simulink library "sm_rollerV_lib_terrain_contact_r9"  (R2026a)
settings: Solver=VariableStepAuto
undefined symbols (not defined in the file): B1, B2, B3, B4, B5, B6, B7, B8, P1, P2, P3, P4, P5, P6, P7, P8, P9, Road, Scene, X, Y, Z
libraries: $bdroot x19, sm_trackV_lib_terrain_contact_elem x18, sm_excv_scene_lib x4, sm_lib x4
Description:
  | Copyright 2024-2026 The MathWorks, Inc.
settings Model: Creator=smiller  LastModifiedBy=smiller

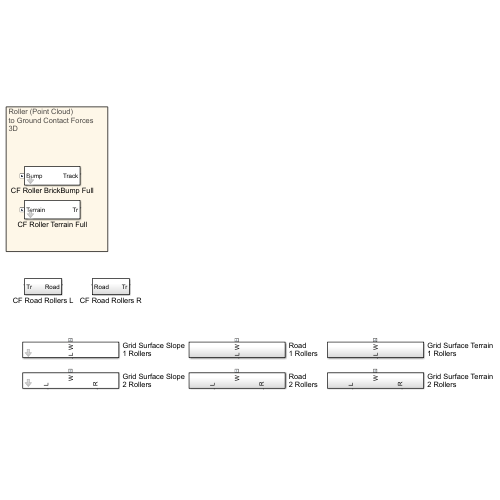
[thumbnail: Simulink's stored preview of the top-level diagram]
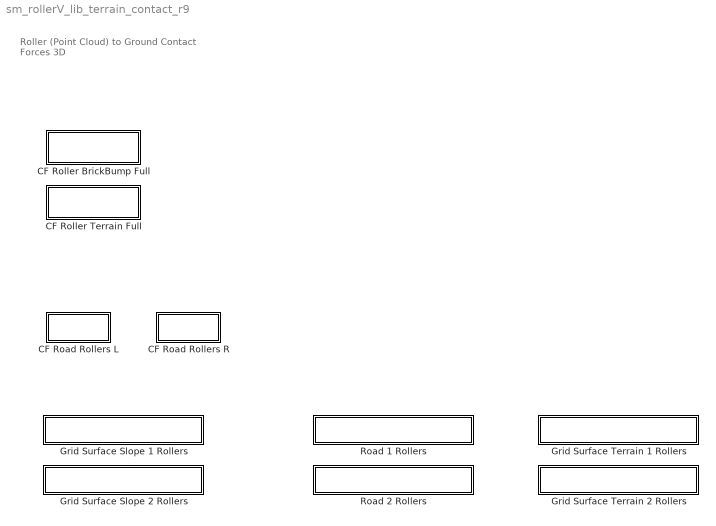
== system sm_rollerV_lib_terrain_contact_r9 ==
  note: Roller (Point Cloud)
      | to Ground Contact Forces
      | 3D
  CF Road Rollers L : Subsystem
  CF Road Rollers R : Subsystem
  CF Roller BrickBump Full : Subsystem  mask(Contact Forces, Rollers to Bump){K_BrickBump=Scene.Contact.BrickBump.K, B_BrickBump=Scene.Contact.BrickBump.B, TW_BrickBump=Scene.Contact.BrickBump.TW}
      mask prompts: K_BrickBump "Normal Stiffness (N/m)"; B_BrickBump "Normal Damping (N/(m/s))"; TW_BrickBump "Normal Transition Width (m)"
      mask help: Models contact force between rolling elements and bump.
  CF Roller Terrain Full : Subsystem  mask(Contact Forces, Rollers to Terrain){K_Road=Scene.Contact.Terrain.K, B_Road=Scene.Contact.Terrain.B, TW_Road=Scene.Contact.Terrain.TW, F_dyn_Road=Scene.Contact.Terrain.mud, F_stat_Road=Scene.Contact.Terrain.mus, CV_Road=Scene.Contact.Terrain.CV}
      mask prompts: K_Road "Normal Stiffness (N/m)"; B_Road "Normal Damping (N/(m/s))"; TW_Road "Normal Transition Width (m)"; F_dyn_Road "Coefficient of Dynamic Friction"; F_stat_Road "Coefficient of Static Friction"; CV_Road "Critical Velocity (m/s)"
      mask help: Models contact force between rolling elements and terrain.
  Grid Surface Slope 1 Rollers : Subsystem  mask{road_len=Scene.Slope.road_len, road_wid=Scene.Slope.road_wid, slope_rise=Scene.Slope.slope_rise, slope_run=Scene.Slope.slope_run, slope_x0=Scene.Slope.slope_start, slope_xres=Scene.Slope.slope_xres, surface_clr=Scene.Slope.clr, surface_opc=Scene.Slope.opc, K_Road=Scene.Contact.Terrain.K, B_Road=Scene.Contact.Terrain.B, TW_Road=Scene.Contact.Terrain.TW, F_dyn_Road=Scene.Contact.Terrain.mud, F_stat_Road=Scene.Contact.Terrain.mus, CV_Road=Scene.Contact.Terrain.CV}
      mask prompts: road_len "Road Length (m)"; road_wid "Road Width (m)"; slope_rise "Slope Rise (m)"; slope_run "Slope Run(m)"; slope_x0 "Slope Start (m)"; slope_xres "Slope Resolution (m)"; surface_clr "Color [R G B] (0-1)"; surface_opc "Opacity (0-1)"; K_Road "Normal Stiffness (N/m)"; B_Road "Normal Damping (N/(m/s))"; TW_Road "Normal Transition Width (m)"; F_dyn_Road "Coefficient of Dynamic Friction"; F_stat_Road "Coefficient of Static Friction"; CV_Road "Critical Velocity (m/s)"
      mask TypeOptions road_len:
      | Grid Surface
      | Slope/road_len
      mask TypeOptions road_wid:
      | Grid Surface
      | Slope/road_wid
      mask TypeOptions slope_rise:
      | Grid Surface
      | Slope/slope_rise
      mask TypeOptions slope_run:
      | Grid Surface
      | Slope/slope_run
      mask TypeOptions slope_x0:
      | Grid Surface
      | Slope/slope_x0
      mask TypeOptions slope_xres:
      | Grid Surface
      | Slope/slope_xres
      mask TypeOptions surface_clr:
      | Grid Surface
      | Slope/surface_clr
      mask TypeOptions surface_opc:
      | Grid Surface
      | Slope/surface_opc
      mask TypeOptions K_Road: CF Track Terrain L/K_Road
      mask TypeOptions B_Road: CF Track Terrain L/B_Road
      mask TypeOptions TW_Road: CF Track Terrain L/TW_Road
      mask TypeOptions F_dyn_Road: CF Track Terrain L/F_dyn_Road
      mask TypeOptions F_stat_Road: CF Track Terrain L/F_stat_Road
      mask TypeOptions CV_Road: CF Track Terrain L/CV_Road
      mask DialogControl cont_slope Prompt: Slope
      mask DialogControl cont_contact Prompt: Contact
  Grid Surface Slope 2 Rollers : Subsystem  mask{road_len=Scene.Slope.road_len, road_wid=Scene.Slope.road_wid, slope_rise=Scene.Slope.slope_rise, slope_run=Scene.Slope.slope_run, slope_x0=Scene.Slope.slope_start, slope_xres=Scene.Slope.slope_xres, surface_clr=Scene.Slope.clr, surface_opc=Scene.Slope.opc, K_Road=Scene.Contact.Terrain.K, B_Road=Scene.Contact.Terrain.B, TW_Road=Scene.Contact.Terrain.TW, F_dyn_Road=Scene.Contact.Terrain.mud, F_stat_Road=Scene.Contact.Terrain.mus, CV_Road=Scene.Contact.Terrain.CV}
      mask prompts: road_len "Road Length (m)"; road_wid "Road Width (m)"; slope_rise "Slope Rise (m)"; slope_run "Slope Run(m)"; slope_x0 "Slope Start (m)"; slope_xres "Slope Resolution (m)"; surface_clr "Color [R G B] (0-1)"; surface_opc "Opacity (0-1)"; K_Road "Normal Stiffness (N/m)"; B_Road "Normal Damping (N/(m/s))"; TW_Road "Normal Transition Width (m)"; F_dyn_Road "Coefficient of Dynamic Friction"; F_stat_Road "Coefficient of Static Friction"; CV_Road "Critical Velocity (m/s)"
      mask TypeOptions road_len:
      | Grid Surface
      | Slope/road_len
      mask TypeOptions road_wid:
      | Grid Surface
      | Slope/road_wid
      mask TypeOptions slope_rise:
      | Grid Surface
      | Slope/slope_rise
      mask TypeOptions slope_run:
      | Grid Surface
      | Slope/slope_run
      mask TypeOptions slope_x0:
      | Grid Surface
      | Slope/slope_x0
      mask TypeOptions slope_xres:
      | Grid Surface
      | Slope/slope_xres
      mask TypeOptions surface_clr:
      | Grid Surface
      | Slope/surface_clr
      mask TypeOptions surface_opc:
      | Grid Surface
      | Slope/surface_opc
      mask TypeOptions K_Road: CF Track Terrain L/K_Road
      mask TypeOptions B_Road: CF Track Terrain L/B_Road
      mask TypeOptions TW_Road: CF Track Terrain L/TW_Road
      mask TypeOptions F_dyn_Road: CF Track Terrain L/F_dyn_Road
      mask TypeOptions F_stat_Road: CF Track Terrain L/F_stat_Road
      mask TypeOptions CV_Road: CF Track Terrain L/CV_Road
      mask DialogControl cont_slope Prompt: Slope
      mask DialogControl cont_contact Prompt: Contact
  Grid Surface Terrain 1 Rollers : Subsystem
  Grid Surface Terrain 2 Rollers : Subsystem
  Road 1 Rollers : Subsystem
  Road 2 Rollers : Subsystem

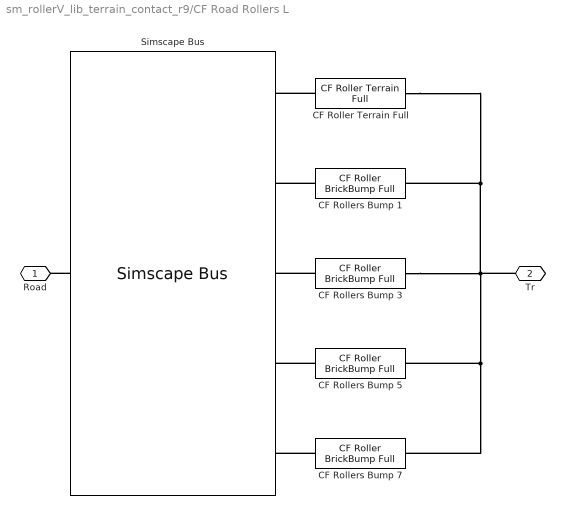
== system sm_rollerV_lib_terrain_contact_r9/CF Road Rollers L ==
  CF Roller Terrain Full : $bdroot/CF Roller Terrain Full  K_Road=Scene.Contact.Terrain.K  B_Road=Scene.Contact.Terrain.B  TW_Road=Scene.Contact.Terrain.TW  F_dyn_Road=Scene.Contact.Terrain.mud  F_stat_Road=Scene.Contact.Terrain.mus  CV_Road=Scene.Contact.Terrain.CV
  "CF Rollers Bump 1 " : $bdroot/CF Roller BrickBump Full  K_BrickBump=Scene.Contact.BrickBump.K  B_BrickBump=Scene.Contact.BrickBump.B  TW_BrickBump=Scene.Contact.BrickBump.TW
  CF Rollers Bump 3 : $bdroot/CF Roller BrickBump Full  K_BrickBump=Scene.Contact.BrickBump.K  B_BrickBump=Scene.Contact.BrickBump.B  TW_BrickBump=Scene.Contact.BrickBump.TW
  CF Rollers Bump 5 : $bdroot/CF Roller BrickBump Full  K_BrickBump=Scene.Contact.BrickBump.K  B_BrickBump=Scene.Contact.BrickBump.B  TW_BrickBump=Scene.Contact.BrickBump.TW
  CF Rollers Bump 7 : $bdroot/CF Roller BrickBump Full  K_BrickBump=Scene.Contact.BrickBump.K  B_BrickBump=Scene.Contact.BrickBump.B  TW_BrickBump=Scene.Contact.BrickBump.TW
  Simscape Bus : SimscapeBus  HierarchyStrings=Road;B1;B3;B5;B7  ConnectionType=Bus: CBO_Road8
  Road : PMIOPort  Side=Left
  Tr : PMIOPort  Port=2  Side=Right
  connections:
  CF Rollers Bump 7/RConn1 -- CF Rollers Bump 5/RConn1 -- "CF Rollers Bump 1 "/RConn1 -- CF Roller Terrain Full/RConn1 -- CF Rollers Bump 3/RConn1 -- Tr/RConn1
  CF Rollers Bump 7/LConn1 -- Simscape Bus/LConn5
  CF Rollers Bump 5/LConn1 -- Simscape Bus/LConn4
  Simscape Bus/RConn1 -- Road/RConn1
  CF Roller Terrain Full/LConn1 -- Simscape Bus/LConn1
  "CF Rollers Bump 1 "/LConn1 -- Simscape Bus/LConn2
  CF Rollers Bump 3/LConn1 -- Simscape Bus/LConn3

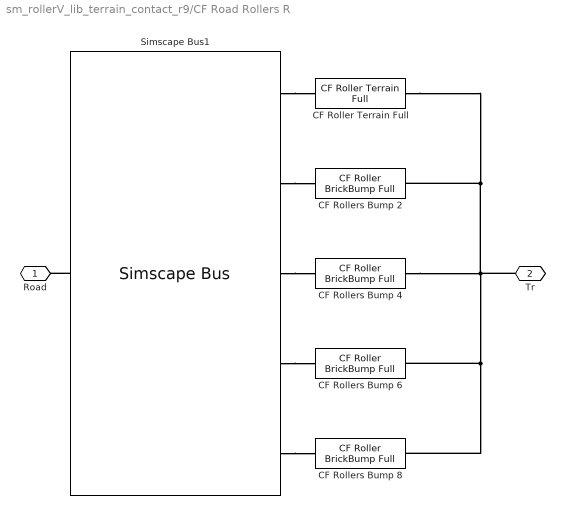
== system sm_rollerV_lib_terrain_contact_r9/CF Road Rollers R ==
  CF Roller Terrain Full : $bdroot/CF Roller Terrain Full  K_Road=Scene.Contact.Terrain.K  B_Road=Scene.Contact.Terrain.B  TW_Road=Scene.Contact.Terrain.TW  F_dyn_Road=Scene.Contact.Terrain.mud  F_stat_Road=Scene.Contact.Terrain.mus  CV_Road=Scene.Contact.Terrain.CV
  "CF Rollers Bump 2 " : $bdroot/CF Roller BrickBump Full  K_BrickBump=Scene.Contact.BrickBump.K  B_BrickBump=Scene.Contact.BrickBump.B  TW_BrickBump=Scene.Contact.BrickBump.TW
  CF Rollers Bump 4 : $bdroot/CF Roller BrickBump Full  K_BrickBump=Scene.Contact.BrickBump.K  B_BrickBump=Scene.Contact.BrickBump.B  TW_BrickBump=Scene.Contact.BrickBump.TW
  CF Rollers Bump 6 : $bdroot/CF Roller BrickBump Full  K_BrickBump=Scene.Contact.BrickBump.K  B_BrickBump=Scene.Contact.BrickBump.B  TW_BrickBump=Scene.Contact.BrickBump.TW
  CF Rollers Bump 8 : $bdroot/CF Roller BrickBump Full  K_BrickBump=Scene.Contact.BrickBump.K  B_BrickBump=Scene.Contact.BrickBump.B  TW_BrickBump=Scene.Contact.BrickBump.TW
  Simscape Bus1 : SimscapeBus  HierarchyStrings=Road;B2;B4;B6;B8  ConnectionType=Bus: CBO_Road8
  Road : PMIOPort  Side=Left
  Tr : PMIOPort  Port=2  Side=Right
  connections:
  Simscape Bus1/LConn3 -- CF Rollers Bump 4/LConn1
  Simscape Bus1/LConn2 -- "CF Rollers Bump 2 "/LConn1
  Simscape Bus1/LConn1 -- CF Roller Terrain Full/LConn1
  Simscape Bus1/RConn1 -- Road/RConn1
  Simscape Bus1/LConn4 -- CF Rollers Bump 6/LConn1
  Simscape Bus1/LConn5 -- CF Rollers Bump 8/LConn1
  CF Rollers Bump 4/RConn1 -- Tr/RConn1 -- CF Rollers Bump 6/RConn1 -- CF Rollers Bump 8/RConn1 -- "CF Rollers Bump 2 "/RConn1 -- CF Roller Terrain Full/RConn1

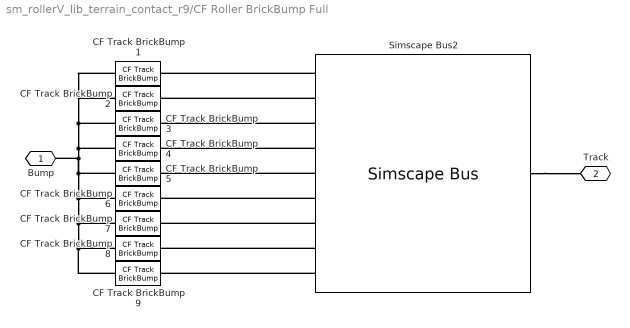
== system sm_rollerV_lib_terrain_contact_r9/CF Roller BrickBump Full ==
  CF Track BrickBump {1..9} (9 alike) : sm_trackV_lib_terrain_contact_elem/CF Track BrickBump  NormalStiffness=K_BrickBump  NormalDamping=B_BrickBump  NormalTransitionRegionWidth=TW_BrickBump
      settings: LibrarySourceBlock=sm_chain_drive_lib/CF_BrickBump
  Simscape Bus2 : SimscapeBus  HierarchyStrings=P1;P2;P3;P4;P5;P6;P7;P8;P9  ConnectionType=Bus: CBO_Roller9
  Bump : PMIOPort  Side=Left
  Track : PMIOPort  Port=2  Side=Right
  connections:
  CF Track BrickBump 6/LConn1 -- CF Track BrickBump 7/LConn1 -- CF Track BrickBump 8/LConn1 -- CF Track BrickBump 9/LConn1 -- Bump/RConn1 -- CF Track BrickBump 1/LConn1 -- CF Track BrickBump 2/LConn1 -- CF Track BrickBump 3/LConn1 -- CF Track BrickBump 4/LConn1 -- CF Track BrickBump 5/LConn1
  Simscape Bus2/RConn1 -- Track/RConn1
  Simscape Bus2/LConn1 -- CF Track BrickBump 1/RConn1
  Simscape Bus2/LConn2 -- CF Track BrickBump 2/RConn1
  Simscape Bus2/LConn4 -- CF Track BrickBump 4/RConn1
  Simscape Bus2/LConn3 -- CF Track BrickBump 3/RConn1
  Simscape Bus2/LConn5 -- CF Track BrickBump 5/RConn1
  Simscape Bus2/LConn6 -- CF Track BrickBump 6/RConn1
  Simscape Bus2/LConn7 -- CF Track BrickBump 7/RConn1
  Simscape Bus2/LConn8 -- CF Track BrickBump 8/RConn1
  Simscape Bus2/LConn9 -- CF Track BrickBump 9/RConn1

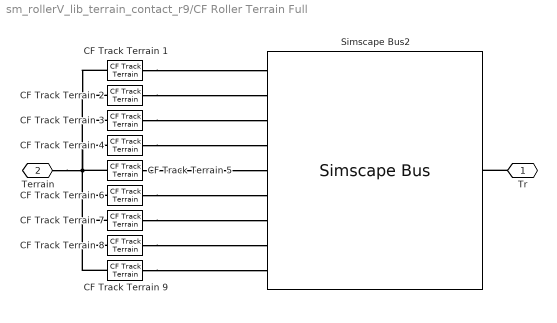
== system sm_rollerV_lib_terrain_contact_r9/CF Roller Terrain Full ==
  CF Track Terrain {1..9} (9 alike) : sm_trackV_lib_terrain_contact_elem/CF Track Terrain  NormalStiffness=K_Road  NormalDamping=B_Road  NormalTransitionRegionWidth=TW_Road  CoefficientOfDynamicFriction=F_dyn_Road  CoefficientOfStaticFriction=F_stat_Road  FrictionalCriticalVelocity=CV_Road
      settings: LibrarySourceBlock=sm_chain_drive_lib/CF_Road
  Simscape Bus2 : SimscapeBus  HierarchyStrings=P1;P2;P3;P4;P5;P6;P7;P8;P9  ConnectionType=Bus: CBO_Roller9
  Tr : PMIOPort  Side=Right
  Terrain : PMIOPort  Port=2  Side=Left
  connections:
  CF Track Terrain 9/RConn1 -- Simscape Bus2/LConn9
  CF Track Terrain 1/LConn1 -- CF Track Terrain 2/LConn1 -- CF Track Terrain 3/LConn1 -- CF Track Terrain 4/LConn1 -- CF Track Terrain 5/LConn1 -- CF Track Terrain 6/LConn1 -- CF Track Terrain 7/LConn1 -- CF Track Terrain 9/LConn1 -- CF Track Terrain 8/LConn1 -- Terrain/RConn1
  CF Track Terrain 8/RConn1 -- Simscape Bus2/LConn8
  CF Track Terrain 3/RConn1 -- Simscape Bus2/LConn3
  CF Track Terrain 2/RConn1 -- Simscape Bus2/LConn2
  CF Track Terrain 1/RConn1 -- Simscape Bus2/LConn1
  CF Track Terrain 7/RConn1 -- Simscape Bus2/LConn7
  CF Track Terrain 5/RConn1 -- Simscape Bus2/LConn5
  CF Track Terrain 4/RConn1 -- Simscape Bus2/LConn4
  CF Track Terrain 6/RConn1 -- Simscape Bus2/LConn6
  Tr/RConn1 -- Simscape Bus2/RConn1

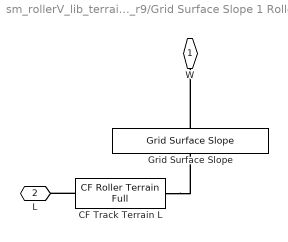
== system sm_rollerV_lib_terrain_contact_r9/Grid Surface Slope 1 Rollers ==
  CF Track Terrain L : $bdroot/CF Roller Terrain Full  K_Road=K_Road  B_Road=B_Road  TW_Road=TW_Road  F_dyn_Road=F_dyn_Road  F_stat_Road=F_stat_Road  CV_Road=CV_Road
  Grid Surface Slope : sm_excv_scene_lib/Grid Surface Slope  road_len=road_len  road_wid=road_wid  slope_run=slope_run  slope_rise=slope_rise  slope_x0=slope_x0  slope_xres=slope_xres  surface_clr=surface_clr  surface_opc=surface_opc
  W : PMIOPort  Side=Right
  L : PMIOPort  Port=2  Side=Left
  connections:
  CF Track Terrain L/RConn1 -- L/RConn1
  Grid Surface Slope/RConn1 -- W/RConn1
  CF Track Terrain L/LConn1 -- Grid Surface Slope/LConn1

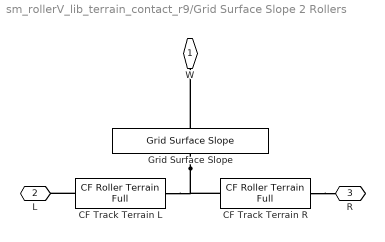
== system sm_rollerV_lib_terrain_contact_r9/Grid Surface Slope 2 Rollers ==
  CF Track Terrain L : $bdroot/CF Roller Terrain Full  K_Road=K_Road  B_Road=B_Road  TW_Road=TW_Road  F_dyn_Road=F_dyn_Road  F_stat_Road=F_stat_Road  CV_Road=CV_Road
  CF Track Terrain R : $bdroot/CF Roller Terrain Full  K_Road=K_Road  B_Road=B_Road  TW_Road=TW_Road  F_dyn_Road=F_dyn_Road  F_stat_Road=F_stat_Road  CV_Road=CV_Road
  Grid Surface Slope : sm_excv_scene_lib/Grid Surface Slope  road_len=road_len  road_wid=road_wid  slope_run=slope_run  slope_rise=slope_rise  slope_x0=slope_x0  slope_xres=slope_xres  surface_clr=surface_clr  surface_opc=surface_opc
  W : PMIOPort  Side=Right
  L : PMIOPort  Port=2  Side=Left
  R : PMIOPort  Port=3  Side=Left
  connections:
  CF Track Terrain R/RConn1 -- R/RConn1
  Grid Surface Slope/LConn1 -- CF Track Terrain R/LConn1 -- CF Track Terrain L/LConn1
  Grid Surface Slope/RConn1 -- W/RConn1
  CF Track Terrain L/RConn1 -- L/RConn1

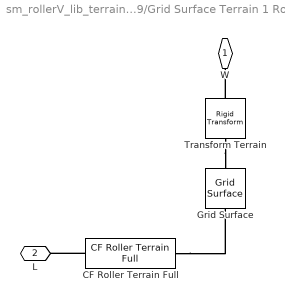
== system sm_rollerV_lib_terrain_contact_r9/Grid Surface Terrain 1 Rollers ==
  CF Roller Terrain Full : $bdroot/CF Roller Terrain Full  K_Road=Scene.Contact.Terrain.K  B_Road=Scene.Contact.Terrain.B  TW_Road=Scene.Contact.Terrain.TW  F_dyn_Road=Scene.Contact.Terrain.mud  F_stat_Road=Scene.Contact.Terrain.mus  CV_Road=Scene.Contact.Terrain.CV
  Grid Surface : sm_lib/Curves and Surfaces/Grid Surface  XGridVector=Scene.Terrain.xg  XGridVectorUnits=m  YGridVector=Scene.Terrain.yg  YGridVectorUnits=m  ZHeights=Scene.Terrain.z_heights_data  ZHeightsUnits=m  GraphicType=FromGeometry  GraphicVisPropType=SimpleVisualProperties  GraphicDiffuseColor=[0.8196 0.7255 0.5098]  GraphicOpacity=1.0  GraphicSpecularColor=[0.5 0.5 0.5 1.0]  GraphicAmbientColor=[0.15 0.15 0.15 1.0]  GraphicEmissiveColor=[0.0 0.0 0.0 1.0]  GraphicShininess=75
  Transform Terrain : sm_lib/Frames and Transforms/Rigid Transform  RotationMethod=None  FollAlignAxisA=+X  BaseAlignAxisA=+Y  FollAlignAxisB=+Y  BaseAlignAxisB=+Z  RotationStandardAxis=+Z  RotationAngle=0.0  RotationAngleUnits=deg  RotationArbitraryAxis=[0 0 1]  RotationSequenceAxes=FollowerAxes  RotationSequence=XYX  RotationSequenceAngles=[0 0 0]  RotationSequenceAnglesUnits=deg  RotationMatrix=[1 0 0; 0 1 0; 0 0 1]  Quaternion=[1 0 0 0]  TranslationMethod=Cartesian  TranslationCartesianOffset="[-45 -45+2.5  -2.75+0.2]"  TranslationCartesianOffsetUnits=m  TranslationStandardAxis=+Z  TranslationStandardOffset=0  TranslationStandardOffsetUnits=m  TranslationROffset=0  TranslationROffsetUnits=m  TranslationThetaOffset=0  TranslationThetaOffsetUnits=deg  TranslationZOffset=0  TranslationZOffsetUnits=m
  W : PMIOPort  Side=Right
  L : PMIOPort  Port=2  Side=Left
  connections:
  CF Roller Terrain Full/RConn1 -- L/RConn1
  Transform Terrain/LConn1 -- W/RConn1
  CF Roller Terrain Full/LConn1 -- Grid Surface/RConn1
  Transform Terrain/RConn1 -- Grid Surface/LConn1

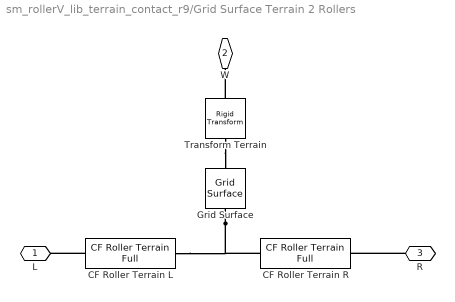
== system sm_rollerV_lib_terrain_contact_r9/Grid Surface Terrain 2 Rollers ==
  CF Roller Terrain L : $bdroot/CF Roller Terrain Full  K_Road=Scene.Contact.Terrain.K  B_Road=Scene.Contact.Terrain.B  TW_Road=Scene.Contact.Terrain.TW  F_dyn_Road=Scene.Contact.Terrain.mud  F_stat_Road=Scene.Contact.Terrain.mus  CV_Road=Scene.Contact.Terrain.CV
  CF Roller Terrain R : $bdroot/CF Roller Terrain Full  K_Road=Scene.Contact.Terrain.K  B_Road=Scene.Contact.Terrain.B  TW_Road=Scene.Contact.Terrain.TW  F_dyn_Road=Scene.Contact.Terrain.mud  F_stat_Road=Scene.Contact.Terrain.mus  CV_Road=Scene.Contact.Terrain.CV
  Grid Surface : sm_lib/Curves and Surfaces/Grid Surface  XGridVector=Scene.Terrain.xg  XGridVectorUnits=m  YGridVector=Scene.Terrain.yg  YGridVectorUnits=m  ZHeights=Scene.Terrain.z_heights_data  ZHeightsUnits=m  GraphicType=FromGeometry  GraphicVisPropType=SimpleVisualProperties  GraphicDiffuseColor=[0.8196 0.7255 0.5098]  GraphicOpacity=1.0  GraphicSpecularColor=[0.5 0.5 0.5 1.0]  GraphicAmbientColor=[0.15 0.15 0.15 1.0]  GraphicEmissiveColor=[0.0 0.0 0.0 1.0]  GraphicShininess=75
  Transform Terrain : sm_lib/Frames and Transforms/Rigid Transform  RotationMethod=None  FollAlignAxisA=+X  BaseAlignAxisA=+Y  FollAlignAxisB=+Y  BaseAlignAxisB=+Z  RotationStandardAxis=+Z  RotationAngle=0.0  RotationAngleUnits=deg  RotationArbitraryAxis=[0 0 1]  RotationSequenceAxes=FollowerAxes  RotationSequence=XYX  RotationSequenceAngles=[0 0 0]  RotationSequenceAnglesUnits=deg  RotationMatrix=[1 0 0; 0 1 0; 0 0 1]  Quaternion=[1 0 0 0]  TranslationMethod=Cartesian  TranslationCartesianOffset="[-45 -45+2.5  -2.75+0.2]"  TranslationCartesianOffsetUnits=m  TranslationStandardAxis=+Z  TranslationStandardOffset=0  TranslationStandardOffsetUnits=m  TranslationROffset=0  TranslationROffsetUnits=m  TranslationThetaOffset=0  TranslationThetaOffsetUnits=deg  TranslationZOffset=0  TranslationZOffsetUnits=m
  L : PMIOPort  Side=Left
  W : PMIOPort  Port=2  Side=Right
  R : PMIOPort  Port=3  Side=Left
  connections:
  R/RConn1 -- CF Roller Terrain R/RConn1
  Transform Terrain/RConn1 -- Grid Surface/LConn1
  Grid Surface/RConn1 -- CF Roller Terrain R/LConn1 -- CF Roller Terrain L/LConn1
  Transform Terrain/LConn1 -- W/RConn1
  CF Roller Terrain L/RConn1 -- L/RConn1

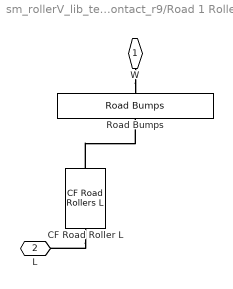
== system sm_rollerV_lib_terrain_contact_r9/Road 1 Rollers ==
  CF Road Roller L : $bdroot/CF Road Rollers L  SystemSampleTime=-1  VariantActivationTime=update diagram  EmptyChoice=off  PassThrough=off  PassThroughVariantControl=(default)  EmptyChoiceVariantControl=(default)  AllowFlexibleInterface=on  Latency=0  AutoFrameSizeCalculation=off
      settings: LibrarySourceBlock=|
      | sm_excv_scene_lib/CF
      | Road
      | Roller L
  Road Bumps : sm_excv_scene_lib/Road Bumps  road_x=Scene.Road.len  road_y=Scene.Road.wid  road_z=Scene.Road.hgt  bump_x=Scene.Road.Bump.len  bump_y=Scene.Road.Bump.wid  bump_z=Scene.Road.Bump.hgt  bloc_y=Scene.Road.Bump.offsety  bloc_z=Scene.Road.Bump.offsetz  bump_x0=Scene.Road.Bump.startx  bloc_dx=Scene.Road.Bump.deltax
  W : PMIOPort  Side=Right
  L : PMIOPort  Port=2  Side=Left
  connections:
  CF Road Roller L/RConn1 -- L/RConn1
  CF Road Roller L/LConn1 -- Road Bumps/LConn1
  W/RConn1 -- Road Bumps/RConn1

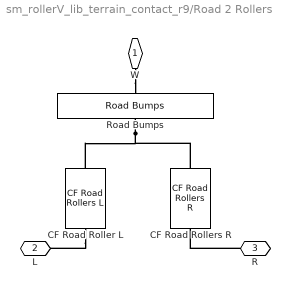
== system sm_rollerV_lib_terrain_contact_r9/Road 2 Rollers ==
  CF Road Roller L : $bdroot/CF Road Rollers L  SystemSampleTime=-1  VariantActivationTime=update diagram  EmptyChoice=off  PassThrough=off  PassThroughVariantControl=(default)  EmptyChoiceVariantControl=(default)  AllowFlexibleInterface=on  Latency=0  AutoFrameSizeCalculation=off
      settings: LibrarySourceBlock=|
      | sm_excv_scene_lib/CF
      | Road
      | Roller L
  CF Road Rollers R : $bdroot/CF Road Rollers R  SystemSampleTime=-1  VariantActivationTime=update diagram  EmptyChoice=off  PassThrough=off  PassThroughVariantControl=(default)  EmptyChoiceVariantControl=(default)  AllowFlexibleInterface=on  Latency=0  AutoFrameSizeCalculation=off
      settings: LibrarySourceBlock=|
      | sm_excv_scene_lib/CF
      | Road
      | Rollers R
  Road Bumps : sm_excv_scene_lib/Road Bumps  road_x=Scene.Road.len  road_y=Scene.Road.wid  road_z=Scene.Road.hgt  bump_x=Scene.Road.Bump.len  bump_y=Scene.Road.Bump.wid  bump_z=Scene.Road.Bump.hgt  bloc_y=Scene.Road.Bump.offsety  bloc_z=Scene.Road.Bump.offsetz  bump_x0=Scene.Road.Bump.startx  bloc_dx=Scene.Road.Bump.deltax
  W : PMIOPort  Side=Right
  L : PMIOPort  Port=2  Side=Left
  R : PMIOPort  Port=3  Side=Left
  connections:
  R/RConn1 -- CF Road Rollers R/RConn1
  W/RConn1 -- Road Bumps/RConn1
  Road Bumps/LConn1 -- CF Road Rollers R/LConn1 -- CF Road Roller L/LConn1
  CF Road Roller L/RConn1 -- L/RConn1
